simulink model "tp1_3"  (R2023b)
settings: Solver=VariableStepAuto  StartTime=0.0  StopTime=50  RelTol=1e-3
settings Model: Creator=rusha  LastModifiedBy=rusha

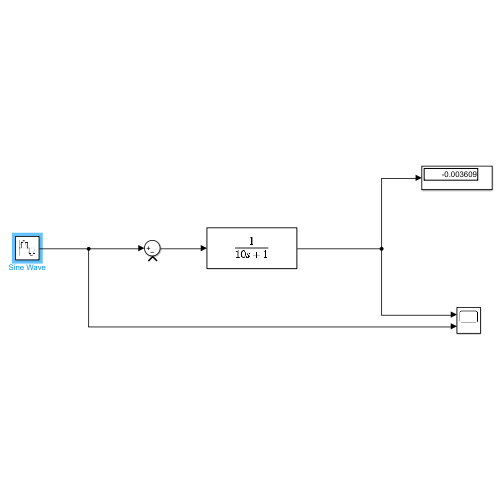
[thumbnail: Simulink's stored preview of the top-level diagram]
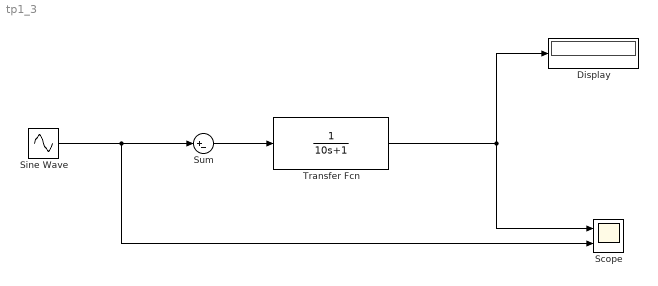
== system tp1_3 ==
  Display : Display
  Scope : Scope  NumInputPorts=2
  Sine Wave : Sin  Frequency=10  SampleTime=0.0001
  Sum : Sum  Inputs=|+-
  Transfer Fcn : TransferFcn  Denominator=[10 1]
  wires:
  Sine Wave/1 -> Scope/2, Sum/1
  Transfer Fcn/1 -> Display/1, Scope/1
  Sum/1 -> Transfer Fcn/1
